simulink model "asbdhc2"  (Simulink 8.0)
settings: Solver=ode45  StartTime=0.0  StopTime=1000  MaxStep=1/30  RelTol=1e-2  AbsTol=1e-3
PreLoadFcn:
  | load asbdhc2_init;
values from neighbouring files (symbols this model uses):
  beaver_b = 14.63    [beaver_4_14_2013.mat]    (also in modelScript.m = 1.4224; monteCarloSim01.mat = 1.4224; simData_12_10_2013.mat = 1.4224; simData_12_9_2013.mat = 1.4224)
  beaver_c = 1.5875    [beaver_4_14_2013.mat]    (also in modelScript.m = 0.3302; monteCarloSim01.mat = 0.3302; simData_12_10_2013.mat = 0.3302; simData_12_9_2013.mat = 0.3302)
  beaver_init_p = 0    [beaver_4_14_2013.mat]    (also in monteCarloSim01.mat; simData_12_10_2013.mat; simData_12_9_2013.mat; simData_4_23_2013.mat)
  beaver_init_pitch = 0.13029612885    [beaver_4_14_2013.mat]    (also in monteCarloSim01.mat; simData_12_10_2013.mat; simData_12_9_2013.mat; simData_4_23_2013.mat)
  beaver_init_q = 0    [beaver_4_14_2013.mat]    (also in monteCarloSim01.mat; simData_12_10_2013.mat; simData_12_9_2013.mat; simData_4_23_2013.mat)
  beaver_init_r = 0    [beaver_4_14_2013.mat]    (also in monteCarloSim01.mat; simData_12_10_2013.mat; simData_12_9_2013.mat; simData_4_23_2013.mat)
  beaver_init_roll = 0    [beaver_4_14_2013.mat]    (also in monteCarloSim01.mat; simData_12_10_2013.mat; simData_12_9_2013.mat; simData_4_23_2013.mat)
  beaver_mass = 2288.231    [beaver_4_14_2013.mat]    (also in modelScript.m = 1.56; monteCarloSim01.mat = 1.56; simData_12_10_2013.mat = 1.56; simData_12_9_2013.mat = 1.56)
  beaver_S = 23.23    [beaver_4_14_2013.mat]    (also in modelScript.m = 0.2589; monteCarloSim01.mat = 0.2589; simData_12_10_2013.mat = 0.2589; simData_12_9_2013.mat = 0.2589)
  CD0 = 0.03    [modelScript.m]    (also in monteCarloSim01.mat; polarFun.m = x(1); simData_12_10_2013.mat; simData_12_9_2013.mat)
  Cl0 = 0.000591    [beaver_4_14_2013.mat]    (also in monteCarloSim01.mat; simData_12_10_2013.mat; simData_12_9_2013.mat; simData_4_23_2013.mat)
  Cl_alpha2_dpt = -0.01406    [beaver_4_14_2013.mat]    (also in monteCarloSim01.mat; simData_12_10_2013.mat; simData_12_9_2013.mat; simData_4_23_2013.mat)
  Cl_beta = -0.0618    [beaver_4_14_2013.mat]    (also in monteCarloSim01.mat; simData_12_10_2013.mat; simData_12_9_2013.mat; simData_4_23_2013.mat)
  Cl_da = -0.09917    [beaver_4_14_2013.mat]    (also in monteCarloSim01.mat; simData_12_10_2013.mat; simData_12_9_2013.mat; simData_4_23_2013.mat)
  Cl_da_alpha = -0.08269    [beaver_4_14_2013.mat]    (also in monteCarloSim01.mat; simData_12_10_2013.mat; simData_12_9_2013.mat; simData_4_23_2013.mat)
  Cl_dr = 0.006934    [beaver_4_14_2013.mat]    (also in monteCarloSim01.mat; simData_12_10_2013.mat; simData_12_9_2013.mat; simData_4_23_2013.mat)
  Cl_p = -0.5045    [beaver_4_14_2013.mat]    (also in monteCarloSim01.mat; simData_12_10_2013.mat; simData_12_9_2013.mat; simData_4_23_2013.mat)
  Cl_r = 0.1695    [beaver_4_14_2013.mat]    (also in monteCarloSim01.mat; simData_12_10_2013.mat; simData_12_9_2013.mat; simData_4_23_2013.mat)
  Cm0 = 0.09448    [beaver_4_14_2013.mat]    (also in monteCarloSim01.mat; simData_12_10_2013.mat; simData_12_9_2013.mat; simData_4_23_2013.mat)
  Cm_alpha = -0.6028    [beaver_4_14_2013.mat]    (also in monteCarloSim01.mat; simData_12_10_2013.mat; simData_12_9_2013.mat; simData_4_23_2013.mat)
  Cm_alpha2 = -2.14    [beaver_4_14_2013.mat]    (also in monteCarloSim01.mat; simData_12_10_2013.mat; simData_12_9_2013.mat; simData_4_23_2013.mat)
  Cm_beta2 = 0.6921    [beaver_4_14_2013.mat]    (also in monteCarloSim01.mat; simData_12_10_2013.mat; simData_12_9_2013.mat; simData_4_23_2013.mat)
  Cm_de = -1.921    [beaver_4_14_2013.mat]    (also in monteCarloSim01.mat; simData_12_10_2013.mat; simData_12_9_2013.mat; simData_4_23_2013.mat)
  Cm_df = 0.4072    [beaver_4_14_2013.mat]    (also in monteCarloSim01.mat; simData_12_10_2013.mat; simData_12_9_2013.mat; simData_4_23_2013.mat)
  Cm_dpt = -0.07895    [beaver_4_14_2013.mat]    (also in monteCarloSim01.mat; simData_12_10_2013.mat; simData_12_9_2013.mat; simData_4_23_2013.mat)
  Cm_q = -15.56    [beaver_4_14_2013.mat]    (also in monteCarloSim01.mat; simData_12_10_2013.mat; simData_12_9_2013.mat; simData_4_23_2013.mat)
  Cm_r = -0.3118    [beaver_4_14_2013.mat]    (also in monteCarloSim01.mat; simData_12_10_2013.mat; simData_12_9_2013.mat; simData_4_23_2013.mat)
  Cn0 = -0.003117    [beaver_4_14_2013.mat]    (also in monteCarloSim01.mat; simData_12_10_2013.mat; simData_12_9_2013.mat; simData_4_23_2013.mat)
  Cn_beta = 0.006719    [beaver_4_14_2013.mat]    (also in monteCarloSim01.mat; simData_12_10_2013.mat; simData_12_9_2013.mat; simData_4_23_2013.mat)
  Cn_beta3 = 0.1373    [beaver_4_14_2013.mat]    (also in monteCarloSim01.mat; simData_12_10_2013.mat; simData_12_9_2013.mat; simData_4_23_2013.mat)
  Cn_da = -0.003872    [beaver_4_14_2013.mat]    (also in monteCarloSim01.mat; simData_12_10_2013.mat; simData_12_9_2013.mat; simData_4_23_2013.mat)
  Cn_dpt3 = -0.003026    [beaver_4_14_2013.mat]    (also in monteCarloSim01.mat; simData_12_10_2013.mat; simData_12_9_2013.mat; simData_4_23_2013.mat)
  Cn_dr = -0.08265    [beaver_4_14_2013.mat]    (also in monteCarloSim01.mat; simData_12_10_2013.mat; simData_12_9_2013.mat; simData_4_23_2013.mat)
  Cn_p = -0.1585    [beaver_4_14_2013.mat]    (also in monteCarloSim01.mat; simData_12_10_2013.mat; simData_12_9_2013.mat; simData_4_23_2013.mat)
  Cn_q = 0.1595    [beaver_4_14_2013.mat]    (also in monteCarloSim01.mat; simData_12_10_2013.mat; simData_12_9_2013.mat; simData_4_23_2013.mat)
  Cn_r = -0.1112    [beaver_4_14_2013.mat]    (also in monteCarloSim01.mat; simData_12_10_2013.mat; simData_12_9_2013.mat; simData_4_23_2013.mat)
  Cx0 = -0.03554    [beaver_4_14_2013.mat]    (also in modelScript.m = 0; monteCarloSim01.mat = 0; simData_12_10_2013.mat = 0; simData_12_9_2013.mat = 0)
  Cx_alpha = 0.00292    [beaver_4_14_2013.mat]    (also in modelScript.m = 0; monteCarloSim01.mat = 0; simData_12_10_2013.mat = 0; simData_12_9_2013.mat = 0)
  Cx_alpha2 = 5.459    [beaver_4_14_2013.mat]    (also in modelScript.m = 0; monteCarloSim01.mat = 0; simData_12_10_2013.mat = 0; simData_12_9_2013.mat = 0)
  Cx_alpha3 = -5.162    [beaver_4_14_2013.mat]    (also in modelScript.m = 0; monteCarloSim01.mat = 0; simData_12_10_2013.mat = 0; simData_12_9_2013.mat = 0)
  Cx_df = -0.09447    [beaver_4_14_2013.mat]    (also in modelScript.m = 0; monteCarloSim01.mat = 0; simData_12_10_2013.mat = 0; simData_12_9_2013.mat = 0)
  Cx_df_alpha = 1.106    [beaver_4_14_2013.mat]    (also in modelScript.m = 0; monteCarloSim01.mat = 0; simData_12_10_2013.mat = 0; simData_12_9_2013.mat = 0)
  Cx_dpt = 0.1161    [beaver_4_14_2013.mat]    (also in modelScript.m = 0; monteCarloSim01.mat = 0; simData_12_10_2013.mat = 0; simData_12_9_2013.mat = 0)
  Cx_dpt2_alpha = 0.1453    [beaver_4_14_2013.mat]    (also in modelScript.m = 0; monteCarloSim01.mat = 0; simData_12_10_2013.mat = 0; simData_12_9_2013.mat = 0)
  Cx_dr = 0.03412    [beaver_4_14_2013.mat]    (also in modelScript.m = 0; monteCarloSim01.mat = 0; simData_12_10_2013.mat = 0; simData_12_9_2013.mat = 0)
  Cx_q = -0.6748    [beaver_4_14_2013.mat]    (also in modelScript.m = 0; monteCarloSim01.mat = 0; simData_12_10_2013.mat = 0; simData_12_9_2013.mat = 0)
  Cy0 = -0.002226    [beaver_4_14_2013.mat]    (also in modelScript.m = 0; monteCarloSim01.mat = 0; simData_12_10_2013.mat = 0; simData_12_9_2013.mat = 0)
  Cy_beta = -0.7678    [beaver_4_14_2013.mat]    (also in modelScript.m = 0; monteCarloSim01.mat = 0; simData_12_10_2013.mat = 0; simData_12_9_2013.mat = 0)
  Cy_da = -0.02956    [beaver_4_14_2013.mat]    (also in modelScript.m = 0; monteCarloSim01.mat = 0; simData_12_10_2013.mat = 0; simData_12_9_2013.mat = 0)
  Cy_dr = 0.1158    [beaver_4_14_2013.mat]    (also in modelScript.m = 0; monteCarloSim01.mat = 0; simData_12_10_2013.mat = 0; simData_12_9_2013.mat = 0)
  Cy_dr_alpha = 0.5238    [beaver_4_14_2013.mat]    (also in modelScript.m = 0; monteCarloSim01.mat = 0; simData_12_10_2013.mat = 0; simData_12_9_2013.mat = 0)
  Cy_p = -0.124    [beaver_4_14_2013.mat]    (also in modelScript.m = 0; monteCarloSim01.mat = 0; simData_12_10_2013.mat = 0; simData_12_9_2013.mat = 0)
  Cy_r = 0.3666    [beaver_4_14_2013.mat]    (also in modelScript.m = 0; monteCarloSim01.mat = 0; simData_12_10_2013.mat = 0; simData_12_9_2013.mat = 0)
  Cz0 = -0.05504    [beaver_4_14_2013.mat]    (also in modelScript.m = 0; monteCarloSim01.mat = 0; simData_12_10_2013.mat = 0; simData_12_9_2013.mat = 0)
  Cz_alpha = -5.578    [beaver_4_14_2013.mat]    (also in modelScript.m = 0; monteCarloSim01.mat = 0; simData_12_10_2013.mat = 0; simData_12_9_2013.mat = 0)
  Cz_alpha3 = 3.442    [beaver_4_14_2013.mat]    (also in modelScript.m = 0; monteCarloSim01.mat = 0; simData_12_10_2013.mat = 0; simData_12_9_2013.mat = 0)
  Cz_de = -0.398    [beaver_4_14_2013.mat]    (also in modelScript.m = 0; monteCarloSim01.mat = 0; simData_12_10_2013.mat = 0; simData_12_9_2013.mat = 0)
  Cz_de_beta = -15.93    [beaver_4_14_2013.mat]    (also in modelScript.m = 0; monteCarloSim01.mat = 0; simData_12_10_2013.mat = 0; simData_12_9_2013.mat = 0)
  Cz_df = -1.377    [beaver_4_14_2013.mat]    (also in modelScript.m = 0; monteCarloSim01.mat = 0; simData_12_10_2013.mat = 0; simData_12_9_2013.mat = 0)
  Cz_df_alpha = -1.261    [beaver_4_14_2013.mat]    (also in modelScript.m = 0; monteCarloSim01.mat = 0; simData_12_10_2013.mat = 0; simData_12_9_2013.mat = 0)
  Cz_dpt = -0.1563    [beaver_4_14_2013.mat]    (also in modelScript.m = 0; monteCarloSim01.mat = 0; simData_12_10_2013.mat = 0; simData_12_9_2013.mat = 0)
  Cz_q = -2.988    [beaver_4_14_2013.mat]    (also in modelScript.m = 0; monteCarloSim01.mat = 0; simData_12_10_2013.mat = 0; simData_12_9_2013.mat = 0)
  Ix = .1147    (= 0.1147)    [modelScript.m]    (also in monteCarloSim01.mat; simData_12_10_2013.mat; simData_12_9_2013.mat; simData_4_26_2013.mat)
  Ixz = .0015    (= 0.0015)    [modelScript.m]    (also in monteCarloSim01.mat; simData_12_10_2013.mat; simData_12_9_2013.mat; simData_4_26_2013.mat)
  Iy = .0576    (= 0.0576)    [modelScript.m]    (also in monteCarloSim01.mat; simData_12_10_2013.mat; simData_12_9_2013.mat; simData_4_26_2013.mat)
  Iz = .1712    (= 0.1712)    [modelScript.m]    (also in monteCarloSim01.mat; simData_12_10_2013.mat; simData_12_9_2013.mat; simData_4_26_2013.mat)
  KCL2 = 1/(pi*.7*beaver_b/beaver_c)    [modelScript.m]    (also in monteCarloSim01.mat = 0.0493425392361; polarFun.m = x(2); simData_12_10_2013.mat = 0.0493425392361; simData_12_9_2013.mat = 0.0493425392361)
  m = state.W/g(1)    [plant.m]
  nonLinearCd = [0.025 0.0283582705905 0.0317165411809 0.0350748117714 0.0384330823618 0.0417913529523 0.0451496235427 0.0485078941332 0.0518661647236 0.0552244353141 0.0585827059046 0.061940976495 ... (1000 elements, 1x1000)]    [NACA0012Adam.mat]    (also in monteCarloSim01.mat; simData_12_10_2013.mat; simData_12_9_2013.mat; simData_4_23_2013.mat)
  nonLinearCl = [0 0.0485067508622 0.0970135017244 0.145520252587 0.194027003449 0.240505289572 0.286480266666 0.332455243759 0.378430220853 0.421875006681 0.463843622747 0.505812238814 ... (1000 elements, 1x1000)]    [NACA0012Adam.mat]    (also in monteCarloSim01.mat; simData_12_10_2013.mat; simData_12_9_2013.mat; simData_4_23_2013.mat)
  nonLinearWindAeroAlpha = [-3.14159265359 -3.13530317881 -3.12901370403 -3.12272422924 -3.11643475446 -3.11014527968 -3.1038558049 -3.09756633012 -3.09127685533 -3.08498738055 -3.07869790577 -3.07240843099 ... (1000 elements, 1x1000)]    [NACA0012Adam.mat]    (also in monteCarloSim01.mat; simData_12_10_2013.mat; simData_12_9_2013.mat; simData_4_23_2013.mat)
  q = state.eulerRates(:,2)    [eulerKalman.m]
  r = state.eulerRates(:,3)    [eulerKalman.m]
  sampleVec = [1/1000 0]    [modelScript.m]    (also in monteCarloSim01.mat = [0.0909090909091 0]; simData_12_10_2013.mat = [0.0909090909091 0]; simData_12_9_2013.mat = [0.001 0]; simData_4_26_2013.mat = [0.02 0])
  u0 = 100/3.28    (= 30.487804878)    [modelScript.m]    (also in monteCarloSim01.mat; simData_12_10_2013.mat; simData_12_9_2013.mat; simData_4_26_2013.mat)
  uaero0 = [-0.0317656979071 -0.0320210159663 -0.0365180369264 0]    [beaver_4_14_2013.mat]    (also in monteCarloSim01.mat; simData_12_10_2013.mat; simData_12_9_2013.mat; simData_4_23_2013.mat)
  v0 = 0    [modelScript.m]    (also in monteCarloSim01.mat; simData_12_10_2013.mat; simData_12_9_2013.mat; simData_4_26_2013.mat)
  w0 = 0    [modelScript.m]    (also in monteCarloSim01.mat; simData_12_10_2013.mat; simData_12_9_2013.mat; simData_4_26_2013.mat)
undefined symbols (not defined in the file or in its folder): Earth, F, Light, MIL, s, sigbuilder_block, WGS84
libraries: aerolibconvert2 x5, aerolibtransform2 x4, aerolibadynsys x3, aerolibasang x3, aerolibwind2 x3, aerolibfltsims x3, aerolibanimutils x2, aerolib6dof2 x1, aerolibnav x1, aerolibutil x1, aerolibatmos2 x1, aerolibgravity2 x1
(part 1 of 2)
Description:
  | Fly the DeHavilland Beaver
  | 
  | This demonstration uses a pilot's joystick to allow you to fly the DeHavilland
  | Beaver modeled with Simulink(R), and Aerospace Blockset(TM) software.  This model has been
  | color coded to aid in locating Aerospace Blockset blocks. The red blocks are
  | Aerospace Blockset blocks, the orange blocks are subsystems containing
  | additional Aerospace Blockset blocks and the white blocks are Simulink blocks.
  | 
  | The DeHavilland Beaver model includes the airframe dynamics, including
  | aerodynamics. Effects of the environment are also modeled, such as wind profiles
  | for the landing phase. Visualization for this model is done via an interface to
  | FlightGear, a open source flight simulator package.
  | 
  | The DeHavilland Beaver was first flown in 1947. Today it is still prized by pilots
  | for its reliability and versatility. The DeHavilland Beaver can be operated on wheels,
  | skis or float landing gear.
  | 
  | Speed Max       110 kts
  | Altitude Max 10,000 ft
  | Range Max       400 nm
  | Load                     6 passengers
  | Crew                     1 member
  | 
  | For more information on the FlightGear interface, see the documentation.
settings Model: Creator=The MathWorks Inc.  LastModifiedBy=mufasa  ExtModeTrigMode=oneshot  ExtModeArmWhenConnect=off  ExtModeAutoUpdateStatusClock=off
settings DataIOCC: LimitDataPoints=off  SignalLoggingSaveFormat=ModelDataLogs  SignalLoggingName=sigsOut
settings OptimizationCC: InlineParams=on  InlineInvariantSignals=on  InitFltsAndDblsToZero=on  EfficientFloat2IntCast=on  EfficientMapNaN2IntZero=off
settings DebuggingCC: SolverPrmCheckMsg=none  MultiTaskDSMMsg=warning  MultiTaskCondExecSysMsg=none  SigSpecEnsureSampleTimeMsg=none  IntegerOverflowMsg=none  FcnCallInpInsideContextMsg=UseLocalSettings
settings HardwareCC: TargetEndianess=LittleEndian  TargetHWDeviceType=MATLAB Host  ProdEqTarget=off
settings RTWCC: IncludeERTFirstTime=on
settings GRTTargetCC: TargetFcnLib=ansi_tfl_tmw.mat  CombineOutputUpdateFcns=off  GRTInterface=on

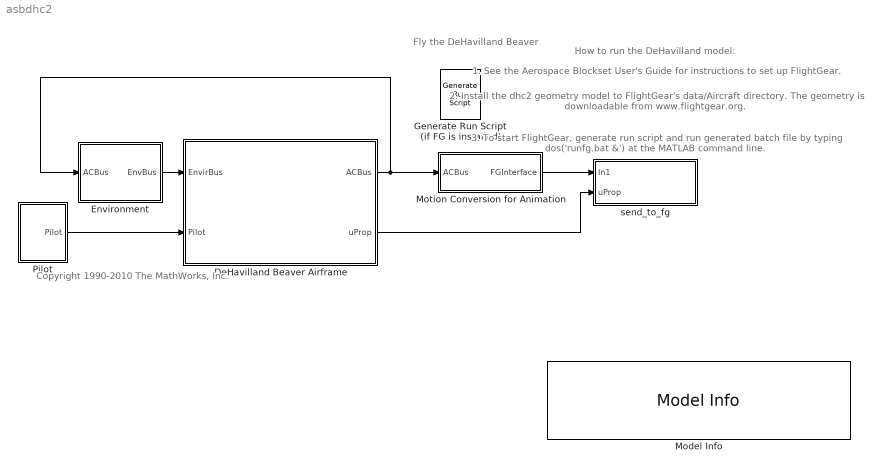
== system asbdhc2 ==
  note: 1. See the Aerospace Blockset User's Guide for instructions
      |     to set up FlightGear.
  note: Copyright 1990-2010 The MathWorks, Inc.
  note: Fly the DeHavilland Beaver
  note: 2. Install the dhc2 geometry model to FlightGear's data/Aircraft
      |     directory. The geometry is downloadable from www.flightgear.org.
  note: 3. To start FlightGear, generate run script and run generated batch
      |     file by typing dos('runfg.bat &') at the MATLAB command line.
  note: How to run the DeHavilland model:
  DeHavilland Beaver Airframe : Subsystem
      mask Display: image(imread('asbbeaver.jpg'))
  Environment : Subsystem
  Generate Run Script (if FG is installed) : aerolibfltsims/Generate Run Script  OutputFileName=runfg.bat  FlightGearBaseDirectory=C:\Program Files\FlightGear  GeometryModelName=dhc2F  DestinationPort=5502  OriginAddress=127.0.0.1  OriginPort=5505  LocalAddress=127.0.0.1  AirportId=KSFO  RunwayId=10L  InitialAltitude=7224  InitialHeading=113  OffsetDistance=4.72  OffsetAzimuth=0  GenerateFile=off  Architecture=Default  dataFlow=Send
  Model Info : simulink/Model-Wide Utilities/Model Info  InitialBlockCM=none  BlockCM=none  Frame=on  DisplayStringWithTags=|  HorizontalTextAlignment=Center  LeftAlignmentValue=0.5  SourceBlockDiagram=asbdhc2  TagMaxNumber=20
      | DeHavilland Beaver model 
      | %<ModelVersion>
      | Based on original work created by
      | Marc Rauw for Delft University of Technology 
      | http://www.dutchroll.com
  Motion Conversion for Animation : Subsystem
      mask Display:
      | port_label('input',1,'ACBus')
      | port_label('output',1,'\lambda,L,h,\phi,\theta,\psi','texmode','on')
  Pilot : Subsystem
  send_to_fg : Subsystem
  wires:
  DeHavilland Beaver Airframe/1(ACBus) -> Motion Conversion for Animation/1(ACBus), Environment/1(ACBus)
  Pilot/1(Pilot) -> DeHavilland Beaver Airframe/2(Pilot)
  Environment/1(EnvBus) -> DeHavilland Beaver Airframe/1(EnvirBus)
  Motion Conversion for Animation/1(FGInterface) -> send_to_fg/1(In1)
  DeHavilland Beaver Airframe/2(uProp) -> send_to_fg/2(uProp)

== system asbdhc2/DeHavilland Beaver Airframe ==
  EnvirBus : Inport
  Pilot : Inport  Port=2
  Aircraft Dynamics : Subsystem
  Calculate Parameters : Subsystem
  ACBus : Outport
  uProp : Outport  Port=2
  wires:
  Pilot/1 -> Aircraft Dynamics/1(Pilot)
  Aircraft Dynamics/1(AC Bus) -> Calculate Parameters/2(ACBus), ACBus/1
  EnvirBus/1 -> Aircraft Dynamics/2(EnvirBus), Calculate Parameters/1(EnvirBus)
  Calculate Parameters/1(FltParams) -> Aircraft Dynamics/3(FltParams)
  Aircraft Dynamics/2(uProp) -> uProp/1

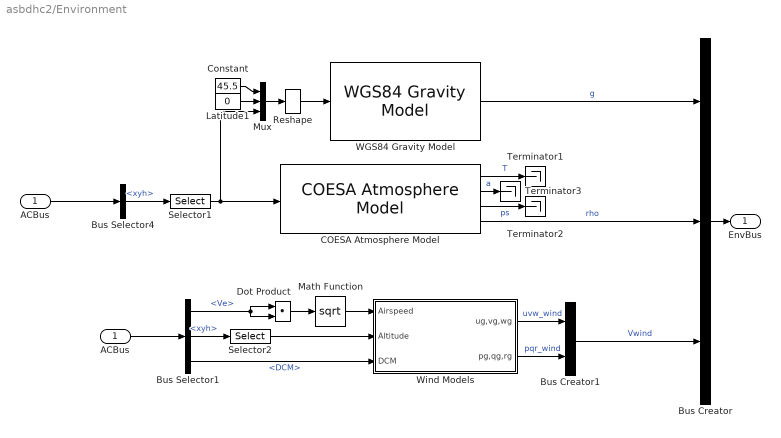
== system asbdhc2/Environment ==
  ACBus : Inport
  "ACBus " : InportShadow
  Bus Creator : BusCreator  Inputs=3
  Bus Creator1 : BusCreator  Inputs=2
  Bus Selector1 : BusSelector  OutputSignals=Ve,xyh,DCM
  Bus Selector4 : BusSelector  OutputSignals=xyh
  COESA Atmosphere Model : aerolibatmos2/COESA Atmosphere Model  units=Metric (MKS)  spec=1976 COESA-extended U.S. Standard Atmosphere  model=Profile  profile_var=High temperature  profile_percent=1%  profile_alt=5 km (16404 ft)  envelope_var=High temperature  envelope_percent=1%  action=Warning
  Constant : Constant  Value=45.5
  Dot Product : DotProduct  InputSameDT=on  OutDataTypeStr=Inherit: Inherit via internal rule
  Latitude1 : Constant  Value=0
  Math Function : Math  Operator=sqrt  SaturateOnIntegerOverflow=on
  Mux : Mux  Inputs=3
  Reshape : Reshape  OutputDimensionality=Row vector (2-D)
  Selector1 : Selector  InputPortWidth=3  IndexOptions=Index vector (dialog)  Indices=[3]  OutputSizes=1
  Selector2 : Selector  InputPortWidth=3  IndexOptions=Index vector (dialog)  Indices=[3]  OutputSizes=1
  Terminator1 : Terminator
  Terminator2 : Terminator
  Terminator3 : Terminator
  "WGS84 Gravity Model " : aerolibgravity2/WGS84 Gravity Model   model=WGS84 Taylor Series  units=Metric (MKS)  no_atmos=on  precessing=on  jd_loc=off  month=October  day=10  year=2004  no_centrifugal=on  action=None
  Wind Models : Subsystem
  EnvBus : Outport
  wires:
  COESA Atmosphere Model/4 -> Bus Creator/2  "rho"
  COESA Atmosphere Model/1 -> Terminator1/1  "T"
  COESA Atmosphere Model/3 -> Terminator2/1  "ps"
  COESA Atmosphere Model/2 -> Terminator3/1  "a"
  Selector1/1 -> COESA Atmosphere Model/1, Mux/3
  Bus Selector1/3 -> Wind Models/3(DCM)  "<DCM>"
  Wind Models/2(pg,qg,rg) -> Bus Creator1/2  "pqr_wind"
  Wind Models/1(ug,vg,wg) -> Bus Creator1/1  "uvw_wind"
  Bus Creator1/1 -> Bus Creator/3  "Vwind"
  Dot Product/1 -> Math Function/1
  Math Function/1 -> Wind Models/1(Airspeed)
  Bus Creator/1 -> EnvBus/1
  ACBus/1 -> Bus Selector4/1
  Bus Selector4/1 -> Selector1/1  "<xyh>"
  "ACBus "/1 -> Bus Selector1/1
  Bus Selector1/2 -> Selector2/1  "<xyh>"
  Selector2/1 -> Wind Models/2(Altitude)
  Bus Selector1/1 -> Dot Product/1, Dot Product/2  "<Ve>"
  Constant/1 -> Mux/1
  Latitude1/1 -> Mux/2
  Mux/1 -> Reshape/1
  "WGS84 Gravity Model "/1 -> Bus Creator/1  "g"
  Reshape/1 -> "WGS84 Gravity Model "/1

== system asbdhc2/Motion Conversion for Animation ==
  ACBus : Inport
  Angle Conversion : aerolibconvert2/Angle Conversion  IU=deg  OU=rad
  Bus Selector : BusSelector  OutputSignals=phi_theta_psi,Hdot,Ve,pqr,Vbody,bodyAccels
  Bus Selector1 : BusSelector  OutputSignals=Xe  OutputAsBus=on
  Constant : Constant  Value=0
  Flat Earth to LLA : aerolibtransform2/Flat Earth to LLA  units=Metric (MKS)  ptype=Earth (WGS84)  F=1/298.257223563  R=6378137  LL0=[37.6272 -122.3896]  psi=0
  Mux : Mux  Inputs=2
  Mux1 : Mux  Inputs=7
  Selector : Selector  InputPortWidth=2  IndexOptions=Index vector (dialog)  Indices=[2 1]  OutputSizes=1
  FGInterface : Outport
  wires:
  Mux1/1 -> FGInterface/1
  Constant/1 -> Flat Earth to LLA/2
  Bus Selector/1 -> Mux1/2  "<phi_theta_psi>"
  Mux/1 -> Mux1/1
  Flat Earth to LLA/2 -> Mux/2
  Flat Earth to LLA/1 -> Angle Conversion/1
  Bus Selector1/1 -> Flat Earth to LLA/1
  ACBus/1 -> Bus Selector/1, Bus Selector1/1
  Selector/1 -> Mux/1
  Bus Selector/2 -> Mux1/3  "<Hdot>"
  Bus Selector/3 -> Mux1/4  "<Ve>"
  Bus Selector/4 -> Mux1/5  "<pqr>"
  Bus Selector/5 -> Mux1/6  "<Vbody>"
  Bus Selector/6 -> Mux1/7  "<bodyAccels>"
  Angle Conversion/1 -> Selector/1

== system asbdhc2/Pilot ==
  Bus Creator : BusCreator  Inputs=2
  Flap : Subsystem  Tag=STV Subsys  LoadFcn=sigbuilder_block('load');  StartFcn=sigbuilder_block('start');  StopFcn=sigbuilder_block('stop');  ClipboardFcn=sigbuilder_block('clipboard');  mask(Sigbuilder block){}
      mask help: Sigbuilder GUI
      mask init:
      | if ~strcmp(get_param(bdroot(gcb),'SimulationStatus'),'stopped') tuvar = sigbuilder_block('maskInit'); end
      settings: CopyFcn=sigbuilder_block('copy');  DeleteFcn=sigbuilder_block('delete');  ModelCloseFcn=sigbuilder_block('modelClose');  PreSaveFcn=sigbuilder_block('preSave');  PauseFcn=sigbuilder_block('pause')  ContinueFcn=sigbuilder_block('continue')  NameChangeFcn=sigbuilder_block('namechange');  OpenFcn=sigbuilder_block('open',[127.5 251.25 511.5 271.5 ]);  CloseFcn=sigbuilder_block('close');
      mask Display: plot(0,0,100,100,[10,10,40,40,10],[80,20,20,80,80],[40,10],[50,50], [40,27,10],[65,72,56],[40,25,25,10],[28,28,43,43]);
  Input Signal  Conditioning : Subsystem
  Mux2 : Mux  Inputs=3
  Pilot Joystick : aerolibanimutils/Pilot Joystick  JoystickID=Joystick1  OutputConfiguration=FourAxis  SampleTime=1/30
  Rate Transition1 : RateTransition  OutPortSampleTime=0
  Rate Transition2 : RateTransition  OutPortSampleTime=0
  Pilot : Outport
  wires:
  Flap/1(Flap) -> Input Signal  Conditioning/3(Flap)
  Rate Transition1/1 -> Input Signal  Conditioning/1(Stick / Throt)
  Rate Transition2/1 -> Input Signal  Conditioning/2(Rudder)
  Input Signal  Conditioning/1(uaero) -> Bus Creator/1  "uaero"
  Input Signal  Conditioning/2(uprop) -> Bus Creator/2  "uprop"
  Bus Creator/1 -> Pilot/1
  Mux2/1 -> Rate Transition1/1
  Pilot Joystick/1 -> Mux2/1
  Pilot Joystick/3 -> Rate Transition2/1
  Pilot Joystick/4 -> Mux2/3
  Pilot Joystick/2 -> Mux2/2

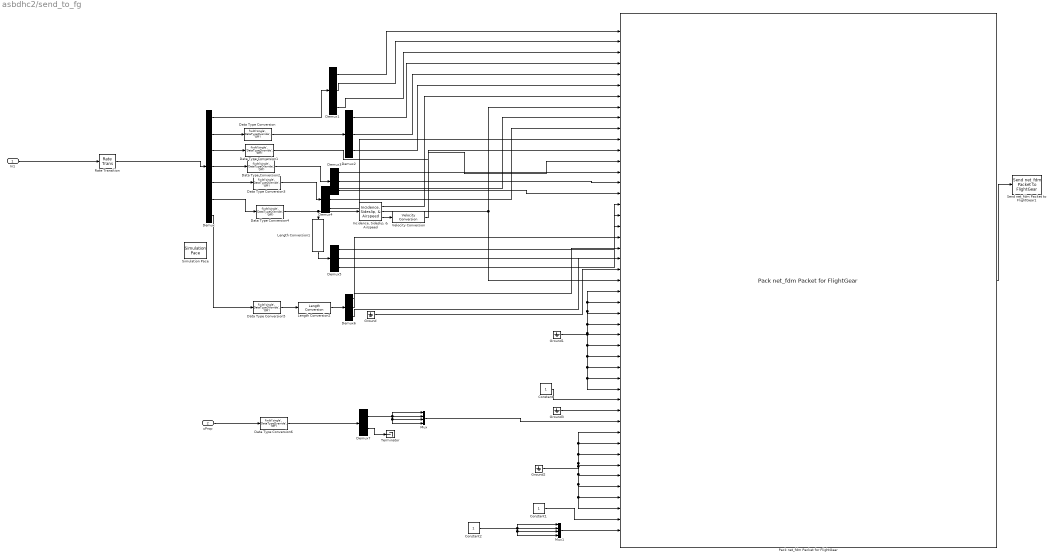
== system asbdhc2/send_to_fg ==
  In1 : Inport  OutDataTypeStr=double
  uProp : Inport  Port=2  OutDataTypeStr=double
  Constant : Constant  OutDataTypeStr=uint32
  Constant1 : Constant  OutDataTypeStr=fixdt('uint32', 'DataTypeOverride', 'Off')
  Constant2 : Constant  OutDataTypeStr=single
  Data Type Conversion{,1..6} (7 alike) : DataTypeConversion  OutDataTypeStr=fixdt('single', 'DataTypeOverride', 'Off')
  Demux : Demux  Outputs=7
  Demux{1..6} (6 alike) : Demux  Outputs=3
  Demux7 : Demux  Outputs=2
  Ground{,1..3} (4 alike) : Ground
  "Incidence, Sideslip, & Airspeed" : aerolibasang/Incidence, Sideslip, & Airspeed
  Length Conversion1 : aerolibconvert2/Length Conversion  IU=m  OU=ft
  Length Conversion2 : aerolibconvert2/Length Conversion  IU=m  OU=ft
  Mux : Mux
  Mux1 : Mux
  Pack net_fdm Packet for FlightGear : aerolibfltsims/Pack net_fdm Packet for FlightGear  FlightGearVersion=v2.0  ShowPositionAttitudeInputs=on  ShowVelocityAccelerationInputs=on  ShowControlSurfacePositionInputs=on  ShowEngineFuelInputs=on  ShowLandingGearInputs=off  ShowEnvironmentInputs=off  SampleTime=1/30
  Rate Transition : RateTransition  Integrity=off  Deterministic=off  OutPortSampleTime=1/30
  Send net_fdm Packet to FlightGear1 : aerolibfltsims/Send net_fdm Packet to FlightGear  DestinationIpAddress=127.0.0.1  DestinationPort=5502  LocalIpPort=-1  varLen=off  SampleTime=1/30
  Simulation Pace : aerolibanimutils/Simulation Pace  SimulationPace=1  SleepMode=MATLAB Thread  OutputPaceError=off  SampleTime=1/30
      settings: AttributesFormatString=%<SimulationPace> sec/sec
  Terminator : Terminator
  Velocity Conversion : aerolibconvert2/Velocity Conversion  IU=m/s  OU=kts
  wires:
  In1/1 -> Rate Transition/1
  Demux/1 -> Demux1/1
  Demux1/1 -> Pack net_fdm Packet for FlightGear/1
  Demux1/2 -> Pack net_fdm Packet for FlightGear/2
  Demux1/3 -> Pack net_fdm Packet for FlightGear/3
  Demux/2 -> Data Type Conversion/1
  Demux2/1 -> Pack net_fdm Packet for FlightGear/4
  Demux2/2 -> Pack net_fdm Packet for FlightGear/5
  Demux2/3 -> Pack net_fdm Packet for FlightGear/6
  Demux/6 -> Data Type Conversion4/1
  "Incidence, Sideslip, & Airspeed"/1 -> Pack net_fdm Packet for FlightGear/7
  "Incidence, Sideslip, & Airspeed"/2 -> Pack net_fdm Packet for FlightGear/8, Pack net_fdm Packet for FlightGear/24
  "Incidence, Sideslip, & Airspeed"/3 -> Velocity Conversion/1
  Demux/4 -> Data Type Conversion2/1
  Demux3/1 -> Pack net_fdm Packet for FlightGear/14
  Demux3/2 -> Pack net_fdm Packet for FlightGear/15
  Demux3/3 -> Pack net_fdm Packet for FlightGear/16
  Demux4/1 -> Pack net_fdm Packet for FlightGear/9
  Demux4/2 -> Pack net_fdm Packet for FlightGear/10
  Demux/5 -> Data Type Conversion3/1
  Ground/1 -> Pack net_fdm Packet for FlightGear/23
  Demux5/1 -> Pack net_fdm Packet for FlightGear/17
  Demux5/2 -> Pack net_fdm Packet for FlightGear/18
  Demux5/3 -> Pack net_fdm Packet for FlightGear/19
  Demux/7 -> Data Type Conversion5/1
  Demux6/1 -> Pack net_fdm Packet for FlightGear/20
  Demux6/2 -> Pack net_fdm Packet for FlightGear/21
  Demux6/3 -> Pack net_fdm Packet for FlightGear/22
  Rate Transition/1 -> Demux/1
  Pack net_fdm Packet for FlightGear/1 -> Send net_fdm Packet to FlightGear1/1
  Demux4/3 -> Pack net_fdm Packet for FlightGear/11
  Demux/3 -> Data Type Conversion1/1
  Data Type Conversion/1 -> Demux2/1
  Data Type Conversion1/1 -> Pack net_fdm Packet for FlightGear/13
  Data Type Conversion2/1 -> Demux3/1
  Data Type Conversion3/1 -> Demux4/1
  Data Type Conversion4/1 -> "Incidence, Sideslip, & Airspeed"/1, Length Conversion1/1
  Data Type Conversion5/1 -> Length Conversion2/1
  Velocity Conversion/1 -> Pack net_fdm Packet for FlightGear/12
  Length Conversion1/1 -> Demux5/1
  Length Conversion2/1 -> Demux6/1
  Ground1/1 -> Pack net_fdm Packet for FlightGear/25, Pack net_fdm Packet for FlightGear/26, Pack net_fdm Packet for FlightGear/27, Pack net_fdm Packet for FlightGear/28, Pack net_fdm Packet for FlightGear/29, Pack net_fdm Packet for FlightGear/30, Pack net_fdm Packet for FlightGear/31, Pack net_fdm Packet for FlightGear/32, Pack net_fdm Packet for FlightGear/33, Pack net_fdm Packet for FlightGear/34
  Constant/1 -> Pack net_fdm Packet for FlightGear/35
  Ground2/1 -> Pack net_fdm Packet for FlightGear/38, Pack net_fdm Packet for FlightGear/39, Pack net_fdm Packet for FlightGear/40, Pack net_fdm Packet for FlightGear/41, Pack net_fdm Packet for FlightGear/42, Pack net_fdm Packet for FlightGear/43, Pack net_fdm Packet for FlightGear/44, Pack net_fdm Packet for FlightGear/45
  Ground3/1 -> Pack net_fdm Packet for FlightGear/36
  uProp/1 -> Data Type Conversion6/1
  Demux7/2 -> Terminator/1
  Demux7/1 -> Mux/1, Mux/2, Mux/3, Mux/4
  Mux/1 -> Pack net_fdm Packet for FlightGear/37
  Constant2/1 -> Mux1/1, Mux1/2, Mux1/3, Mux1/4
  Mux1/1 -> Pack net_fdm Packet for FlightGear/47
  Data Type Conversion6/1 -> Demux7/1
  Constant1/1 -> Pack net_fdm Packet for FlightGear/46

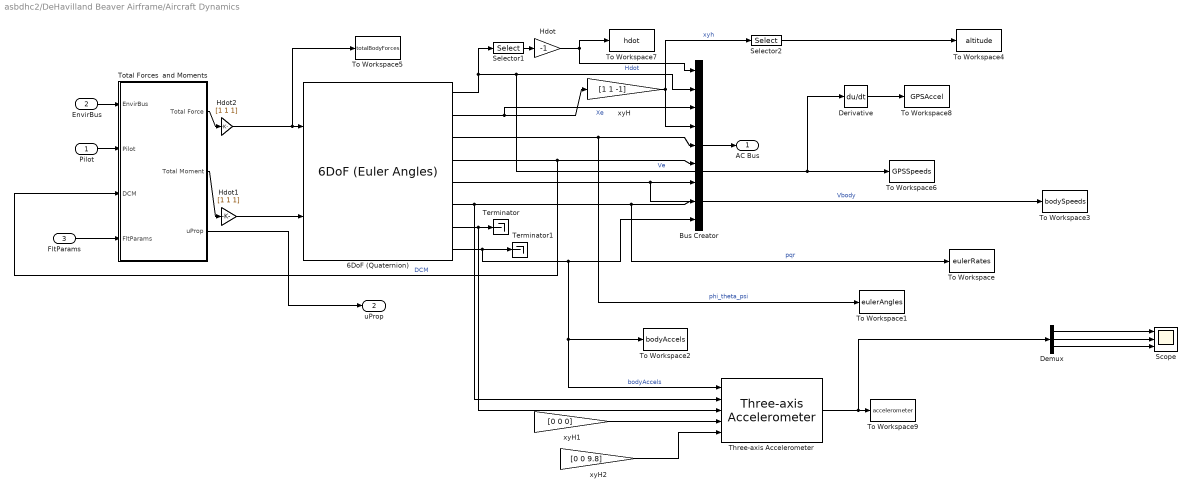
== system asbdhc2/DeHavilland Beaver Airframe/Aircraft Dynamics ==
  Pilot : Inport
  EnvirBus : Inport  Port=2
  FltParams : Inport  Port=3
  6DoF (Quaternion) : aerolib6dof2/6DoF (Euler Angles)  units=Metric (MKS)  mtype=Fixed  rep=Quaternion  xme_0=xme_0  Vm_0=[u0 v0 w0]  eul_0=[beaver_init_roll, beaver_init_pitch, 113/180*pi]  pm_0=[beaver_init_p, beaver_init_q, beaver_init_r]  mass_0=beaver_mass  mass_e=0  mass_f=0  inertia=[Ix 0 Ixz; 0 Iy 0; Ixz 0 Iz]  inertia_e=eye(3)  inertia_f=eye(3)  k_quat=1.0
  Bus Creator : BusCreator  Inputs=9
  Demux : Demux  Outputs=3
  Derivative : Derivative
  Hdot : Gain  Gain=-1  SaturateOnIntegerOverflow=on  OutDataTypeStr=Inherit: Same as input  ParamDataTypeStr=Inherit: Same as input
  Hdot1 : Gain  Gain=[1 1 1]  SaturateOnIntegerOverflow=on  OutDataTypeStr=Inherit: Same as input  ParamDataTypeStr=Inherit: Same as input
  Hdot2 : Gain  Gain=[1 1 1]  SaturateOnIntegerOverflow=on  OutDataTypeStr=Inherit: Same as input  ParamDataTypeStr=Inherit: Same as input
  Scope : Scope  NumInputPorts=3
      settings: TimeRange=10  YMin=-1~-1~-35  YMax=1~1~35
  Selector1 : Selector  InputPortWidth=3  IndexOptions=Index vector (dialog)  Indices=[3]  OutputSizes=1
  Selector2 : Selector  InputPortWidth=3  IndexOptions=Index vector (dialog)  Indices=[3]  OutputSizes=1
  Terminator : Terminator
  Terminator1 : Terminator
  Three-axis Accelerometer : aerolibnav/Three-axis Accelerometer  units=Metric (MKS)  acc=[0 0 0]  gtype=on  dtype_a=on  w_a=190  z_a=0.707  a_sf_cc=[1 0 0; 0 1 0; 0 0 1]  a_bias=[0 0 0]  a_rand=off  a_seeds=[23093 23094 23095]  a_pow=[0.001 0.001 0.001]  a_sat="[-inf  -inf  -inf  inf inf inf]"  a_Ts=0
  To Workspace : ToWorkspace  VariableName=eulerRates  SampleTime=sampleVec  SaveFormat=Structure With Time
  To Workspace1 : ToWorkspace  VariableName=eulerAngles  SampleTime=sampleVec  SaveFormat=Structure With Time
  To Workspace2 : ToWorkspace  VariableName=bodyAccels  SampleTime=sampleVec  SaveFormat=Structure With Time
  To Workspace3 : ToWorkspace  VariableName=bodySpeeds  SampleTime=sampleVec  SaveFormat=Structure With Time
  To Workspace4 : ToWorkspace  VariableName=altitude  SampleTime=-1  SaveFormat=Structure With Time
  To Workspace5 : ToWorkspace  VariableName=totalBodyForces  SampleTime=-1  SaveFormat=Structure With Time
  To Workspace6 : ToWorkspace  VariableName=GPSSpeeds  SampleTime=[1/5 0]  SaveFormat=Structure With Time
  To Workspace7 : ToWorkspace  VariableName=hdot  SampleTime=-1  SaveFormat=Structure With Time
  To Workspace8 : ToWorkspace  VariableName=GPSAccel  SampleTime=[1/50 0]  SaveFormat=Structure With Time
  To Workspace9 : ToWorkspace  VariableName=accelerometer  SampleTime=sampleVec  SaveFormat=Structure With Time
  Total Forces  and Moments : Subsystem
  xyH : Gain  Gain=[1 1 -1]  SaturateOnIntegerOverflow=on  OutDataTypeStr=Inherit: Same as input  ParamDataTypeStr=Inherit: Same as input
  xyH1 : Gain  Gain=[0 0 0]  SaturateOnIntegerOverflow=on  OutDataTypeStr=Inherit: Same as input  ParamDataTypeStr=Inherit: Same as input
  xyH2 : Gain  Gain=[0 0 9.8]  SaturateOnIntegerOverflow=on  OutDataTypeStr=Inherit: Same as input  ParamDataTypeStr=Inherit: Same as input
  AC Bus : Outport
  uProp : Outport  Port=2
  wires:
  6DoF (Quaternion)/4 -> Bus Creator/6, Total Forces  and Moments/3(DCM)  "DCM"
  6DoF (Quaternion)/3 -> Bus Creator/5, To Workspace1/1  "phi_theta_psi"
  6DoF (Quaternion)/2 -> xyH/1, Bus Creator/3  "Xe"
  6DoF (Quaternion)/5 -> Bus Creator/7, To Workspace3/1  "Vbody"
  6DoF (Quaternion)/7 -> Terminator/1, Three-axis Accelerometer/3
  6DoF (Quaternion)/1 -> Selector1/1, Bus Creator/2, To Workspace6/1, Derivative/1  "Ve"
  Pilot/1 -> Total Forces  and Moments/2(Pilot)
  Selector1/1 -> Hdot/1
  Total Forces  and Moments/1(Total Force) -> Hdot2/1
  Total Forces  and Moments/2(Total Moment) -> Hdot1/1
  xyH/1 -> Bus Creator/4, Selector2/1  "xyh"
  Hdot/1 -> Bus Creator/1, To Workspace7/1  "Hdot"
  6DoF (Quaternion)/8 -> Terminator1/1, Bus Creator/9, Three-axis Accelerometer/1, To Workspace2/1  "bodyAccels"
  Bus Creator/1 -> AC Bus/1
  EnvirBus/1 -> Total Forces  and Moments/1(EnvirBus)
  6DoF (Quaternion)/6 -> Three-axis Accelerometer/2, Bus Creator/8, To Workspace/1  "pqr"
  FltParams/1 -> Total Forces  and Moments/4(FltParams)
  Total Forces  and Moments/3(uProp) -> uProp/1
  Selector2/1 -> To Workspace4/1
  Derivative/1 -> To Workspace8/1
  Hdot1/1 -> 6DoF (Quaternion)/2
  Hdot2/1 -> 6DoF (Quaternion)/1, To Workspace5/1
  xyH1/1 -> Three-axis Accelerometer/4
  Demux/1 -> Scope/1
  Demux/2 -> Scope/2
  Demux/3 -> Scope/3
  Three-axis Accelerometer/1 -> Demux/1, To Workspace9/1
  xyH2/1 -> Three-axis Accelerometer/5

== system asbdhc2/DeHavilland Beaver Airframe/Calculate Parameters ==
  EnvirBus : Inport
  ACBus : Inport  Port=2
  "ACBus " : InportShadow  Port=2
  Bus Creator : BusCreator  Inputs=5
  Bus Selector1 : BusSelector  OutputSignals=rho
  Bus Selector2 : BusSelector  OutputSignals=Vbody
  Bus Selector3 : BusSelector  OutputSignals=pqr,Ve
  Bus Selector4 : BusSelector  OutputSignals=Vwind.uvw_wind,Vwind.pqr_wind
  Dynamic Pressure : aerolibasang/Dynamic Pressure
  "Incidence, Sideslip, & Airspeed" : aerolibasang/Incidence, Sideslip, & Airspeed
  Sum2 : Sum  Inputs=|++  SaturateOnIntegerOverflow=on  InputSameDT=on  OutDataTypeStr=Inherit: Same as first input
  Sum4 : Sum  Inputs=+-|  SaturateOnIntegerOverflow=on  InputSameDT=on  OutDataTypeStr=Inherit: Same as first input
  To Workspace : ToWorkspace  VariableName=rho  SampleTime=sampleVec  SaveFormat=Structure With Time
  FltParams : Outport
  wires:
  "ACBus "/1 -> Bus Selector2/1
  Bus Creator/1 -> FltParams/1
  Bus Selector3/1 -> Sum2/2  "<pqr>"
  ACBus/1 -> Bus Selector3/1
  Bus Selector1/1 -> Dynamic Pressure/2, To Workspace/1  "<rho>"
  EnvirBus/1 -> Bus Selector1/1, Bus Selector4/1
  Dynamic Pressure/1 -> Bus Creator/5  "Qdyn"
  Bus Selector3/2 -> Dynamic Pressure/1  "<Ve>"
  Bus Selector4/2 -> Sum2/1  "<pqr_wind>"
  Sum4/1 -> "Incidence, Sideslip, & Airspeed"/1
  "Incidence, Sideslip, & Airspeed"/1 -> Bus Creator/1  "alpha"
  "Incidence, Sideslip, & Airspeed"/2 -> Bus Creator/2  "beta"
  "Incidence, Sideslip, & Airspeed"/3 -> Bus Creator/3  "V"
  Bus Selector2/1 -> Sum4/1  "<Vbody>"
  Bus Selector4/1 -> Sum4/2  "<uvw_wind>"
  Sum2/1 -> Bus Creator/4  "pqr_tot"

== system asbdhc2/Environment/Wind Models ==
  Airspeed : Inport
  Altitude : Inport  Port=2
  DCM : Inport  Port=3
  "DCM " : InportShadow  Port=3
  Discrete Wind Gust Model : aerolibwind2/Discrete Wind Gust Model  units=Metric (MKS)  Gx=off  Gy=off  Gz=off  t_0=20  d_m=[120 120 80]  v_m=[3.5 3.5 3.0]
  Dryden Wind Turbulence Model  (Continuous (+q -r)) : aerolibwind2/Dryden Wind Turbulence Model  (Continuous (+q -r))  units=Metric (MKS)  spec=MIL-F-8785C  model=Continuous Dryden (+q -r)  W20=windSpeed  Wdeg=0  TurbProb=10^-2 - Light  L_high=533.4  Wingspan=beaver_b  ts=0.1  Seed=[23341 23342 23343 23344]  T_on=on
  Sum : Sum  Inputs=+++  SaturateOnIntegerOverflow=on  InputSameDT=on  OutDataTypeStr=Inherit: Same as first input
  Wind Shear Model : aerolibwind2/Wind Shear Model  units=Metric (MKS)  phase=Category C - Terminal Flight Phase  W_20=windSpeed  Wdeg=0
  ug,vg,wg : Outport
  pg,qg,rg : Outport  Port=2
  wires:
  "DCM "/1 -> Dryden Wind Turbulence Model  (Continuous (+q -r))/3
  Wind Shear Model/1 -> Sum/1
  Dryden Wind Turbulence Model  (Continuous (+q -r))/1 -> Sum/2
  Discrete Wind Gust Model/1 -> Sum/3
  Sum/1 -> ug,vg,wg/1
  DCM/1 -> Wind Shear Model/2
  Airspeed/1 -> Dryden Wind Turbulence Model  (Continuous (+q -r))/2, Discrete Wind Gust Model/1
  Dryden Wind Turbulence Model  (Continuous (+q -r))/2 -> pg,qg,rg/1
  Altitude/1 -> Dryden Wind Turbulence Model  (Continuous (+q -r))/1, Wind Shear Model/1

== system asbdhc2/Pilot/Flap ==
  Demux : Demux  Tag=STV Demux  Outputs=1
  FromWs : FromWorkspace  Tag=STV FromWs  VariableName=tuvar  SampleTime=0  OutputAfterFinalValue=Holding final value  SigBuilderData=DataTag0  VnvData=DataTag1
      SigBuilderData=|
      | dataSet.timeRange = [0 300]
      | dataSet.name = 'Group 1'
      | sbobj.Groups.Name = 'Group 1'
      | sbobj.Groups.Signals.Name = 'Flap'
      | sbobj.Groups.Signals.XData = [0 4 4 6 6 300]
      | sbobj.Groups.Signals.YData = [0 0 0 0 0 0]
      | sbobj.Groups.TimeRange = [0 300]
  Flap : Outport  Tag=STV Outport
  wires:
  Demux/1 -> Flap/1
  FromWs/1 -> Demux/1

== system asbdhc2/Pilot/Input Signal  Conditioning ==
  Stick / Throt : Inport
  Rudder : Inport  Port=2
  Flap : Inport  Port=3
  Angle Conversion5 : aerolibconvert2/Angle Conversion  IU=deg  OU=rad
  Look-Up Table : Lookup  InputValues=[0:3]  Table=[0 4 10 20]  SaturateOnIntegerOverflow=on
  Mux1 : Mux
  Mux2 : Mux  Inputs=2
  RPM2ManifoldPressure : Lookup_n-D  NumberOfTableDimensions=1  BreakpointsForDimension1=[0 1800 2300]  IndexSearchMethod=Linear search  BeginIndexSearchUsingPreviousIndexResult=on  Table=[0 22.5735 26]  ExtrapMethod=Clip  InputSameDT=on
  Rate Limiter : RateLimiter  RisingSlewLimit=0.5  FallingSlewLimit=-0.5
  Throttle2RPM : Lookup_n-D  NumberOfTableDimensions=1  BreakpointsForDimension1=(1/6)*(3+([-3:3]))  IndexSearchMethod=Linear search  BeginIndexSearchUsingPreviousIndexResult=on  Table=((1+tanh([-3:3]))/(1+tanh(2.65))-0.0025)*2300  ExtrapMethod=Clip  InputSameDT=on
  demux : Demux  Outputs=3
  flip sign : Gain  Gain=-25  SaturateOnIntegerOverflow=on  OutDataTypeStr=Inherit: Same as input  ParamDataTypeStr=Inherit: Same as input
  flip sign1 : Gain  Gain=-15  SaturateOnIntegerOverflow=on  OutDataTypeStr=Inherit: Same as input  ParamDataTypeStr=Inherit: Same as input
  flip sign2 : Gain  Gain=-20  SaturateOnIntegerOverflow=on  OutDataTypeStr=Inherit: Same as input  ParamDataTypeStr=Inherit: Same as input
  uaero : Outport
  uprop : Outport  Port=2
  wires:
  demux/3 -> Throttle2RPM/1
  Flap/1 -> Rate Limiter/1
  Rate Limiter/1 -> Look-Up Table/1
  Stick / Throt/1 -> demux/1
  Rudder/1 -> flip sign/1
  Look-Up Table/1 -> Mux1/4
  demux/1 -> flip sign1/1
  demux/2 -> flip sign2/1
  Mux1/1 -> Angle Conversion5/1
  Angle Conversion5/1 -> uaero/1
  RPM2ManifoldPressure/1 -> Mux2/2
  Mux2/1 -> uprop/1
  flip sign/1 -> Mux1/3
  Throttle2RPM/1 -> Mux2/1, RPM2ManifoldPressure/1
  flip sign1/1 -> Mux1/2
  flip sign2/1 -> Mux1/1

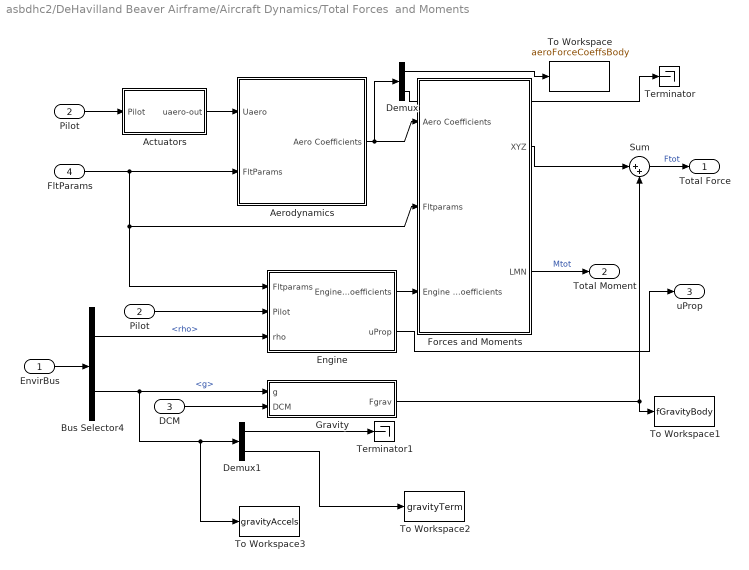
== system asbdhc2/DeHavilland Beaver Airframe/Aircraft Dynamics/Total Forces  and Moments ==
  EnvirBus : Inport
  Pilot : Inport  Port=2
  DCM : Inport  Port=3
  FltParams : Inport  Port=4
  Actuators : Subsystem
  Aerodynamics : Subsystem
  Bus Selector4 : BusSelector  OutputSignals=rho,g
  Demux : Demux  Outputs=[3 3]
  Demux1 : Demux  Outputs=[2 1]
  "Engine " : Subsystem
  Forces and Moments : Subsystem
  "Gravity " : Subsystem
  "Pilot " : InportShadow  Port=2
  Sum : Sum  Inputs=|++  SaturateOnIntegerOverflow=on  InputSameDT=on  OutDataTypeStr=Inherit: Same as first input
  Terminator : Terminator
  Terminator1 : Terminator
  To Workspace : ToWorkspace  VariableName=aeroForceCoeffsBody  SampleTime=-1  SaveFormat=Structure With Time
  To Workspace1 : ToWorkspace  VariableName=fGravityBody  SampleTime=sampleVec  SaveFormat=Structure With Time
  To Workspace2 : ToWorkspace  VariableName=gravityTerm  SampleTime=-1  SaveFormat=Structure With Time
  To Workspace3 : ToWorkspace  VariableName=gravityAccels  SampleTime=sampleVec  SaveFormat=Structure With Time
  Total Force : Outport
  Total Moment : Outport  Port=2
  uProp : Outport  Port=3
  wires:
  Forces and Moments/1(XYZ) -> Sum/1
  "Engine "/1(Engine Coefficients) -> Forces and Moments/3(Engine Coefficients)
  "Gravity "/1(Fgrav) -> Sum/2, To Workspace1/1
  Aerodynamics/1(Aero Coefficients) -> Forces and Moments/1(Aero Coefficients), Demux/1
  Pilot/1 -> Actuators/1(Pilot)
  Bus Selector4/1 -> "Engine "/3(rho)  "<rho>"
  DCM/1 -> "Gravity "/2(DCM)
  Bus Selector4/2 -> "Gravity "/1(g), To Workspace3/1, Demux1/1  "<g>"
  Sum/1 -> Total Force/1  "Ftot"
  Forces and Moments/2(LMN) -> Total Moment/1  "Mtot"
  "Pilot "/1 -> "Engine "/2(Pilot)
  FltParams/1 -> Forces and Moments/2(Fltparams), "Engine "/1(Fltparams), Aerodynamics/2(FltParams)
  Actuators/1(uaero-out) -> Aerodynamics/1(Uaero)
  EnvirBus/1 -> Bus Selector4/1
  "Engine "/2(uProp) -> uProp/1
  Demux/1 -> To Workspace/1
  Demux/2 -> Terminator/1
  Demux1/2 -> To Workspace2/1
  Demux1/1 -> Terminator1/1

== system asbdhc2/DeHavilland Beaver Airframe/Aircraft Dynamics/Total Forces  and Moments/Actuators ==
  Pilot : Inport
  Bus Selector2 : BusSelector  OutputSignals=uaero
  Demux : Demux
  Initial inputs for aero : Constant  Value=uaero0
  Mux : Mux
  Sum1 : Sum  Inputs=++|  SaturateOnIntegerOverflow=on  InputSameDT=on  OutDataTypeStr=Inherit: Same as first input
  uaero-out : Outport
  wires:
  Pilot/1 -> Bus Selector2/1
  Initial inputs for aero/1 -> Sum1/1
  Sum1/1 -> uaero-out/1
  Bus Selector2/1 -> Demux/1  "<uaero>"
  Demux/4 -> Mux/4
  Demux/1 -> Mux/1
  Demux/2 -> Mux/2
  Demux/3 -> Mux/3
  Mux/1 -> Sum1/2

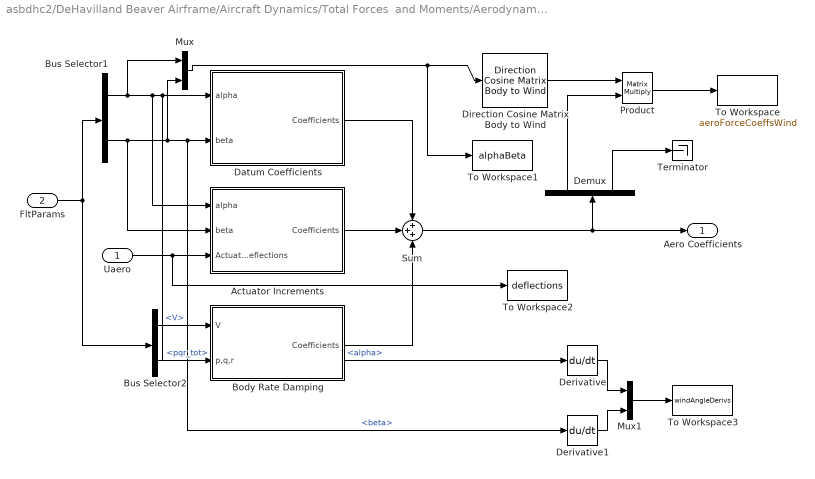
== system asbdhc2/DeHavilland Beaver Airframe/Aircraft Dynamics/Total Forces  and Moments/Aerodynamics ==
  Uaero : Inport
  FltParams : Inport  Port=2
  Actuator Increments : Subsystem
  Body Rate Damping : Subsystem
  Bus Selector1 : BusSelector  OutputSignals=alpha,beta
  Bus Selector2 : BusSelector  OutputSignals=V,pqr_tot
  Datum Coefficients : Subsystem
  Demux : Demux  Outputs=[3 3]
  Derivative : Derivative
  Derivative1 : Derivative
  Direction Cosine Matrix Body to Wind : aerolibtransform2/Direction Cosine Matrix Body to Wind
  Mux : Mux  Inputs=2
  Mux1 : Mux  Inputs=2
  Product : Product  Multiplication=Matrix(*)  RndMeth=Zero
  Sum : Sum  Inputs=+++  SaturateOnIntegerOverflow=on
  Terminator : Terminator
  To Workspace : ToWorkspace  VariableName=aeroForceCoeffsWind  SampleTime=-1  SaveFormat=Structure With Time
  To Workspace1 : ToWorkspace  VariableName=alphaBeta  SampleTime=sampleVec  SaveFormat=Structure
  To Workspace2 : ToWorkspace  VariableName=deflections  SampleTime=-1  SaveFormat=Structure With Time
  To Workspace3 : ToWorkspace  VariableName=windAngleDerivs  SampleTime=sampleVec  SaveFormat=Structure With Time
  Aero Coefficients : Outport
  wires:
  Bus Selector1/2 -> Actuator Increments/2(beta), Datum Coefficients/2(beta), Derivative1/1, Mux/2  "<beta>"
  Sum/1 -> Aero Coefficients/1, Demux/1
  Body Rate Damping/1(Coefficients) -> Sum/3
  Datum Coefficients/1(Coefficients) -> Sum/1
  Actuator Increments/1(Coefficients) -> Sum/2
  Bus Selector2/1 -> Body Rate Damping/1(V)  "<V>"
  Bus Selector2/2 -> Body Rate Damping/2(p,q,r)  "<pqr_tot>"
  Uaero/1 -> Actuator Increments/3(Actuator Deflections), To Workspace2/1
  Bus Selector1/1 -> Actuator Increments/1(alpha), Datum Coefficients/1(alpha), Derivative/1, Mux/1  "<alpha>"
  FltParams/1 -> Bus Selector1/1, Bus Selector2/1
  Mux/1 -> Direction Cosine Matrix Body to Wind/1, To Workspace1/1
  Direction Cosine Matrix Body to Wind/1 -> Product/1
  Product/1 -> To Workspace/1
  Demux/1 -> Product/2
  Demux/2 -> Terminator/1
  Derivative/1 -> Mux1/1
  Derivative1/1 -> Mux1/2
  Mux1/1 -> To Workspace3/1

== system asbdhc2/DeHavilland Beaver Airframe/Aircraft Dynamics/Total Forces  and Moments/Engine  ==
  Fltparams : Inport
  Pilot : Inport  Port=2
  rho : Inport  Port=3
  Bus Selector1 : BusSelector  OutputSignals=uprop
  Bus Selector4 : BusSelector  OutputSignals=V,alpha
  eng : Subsystem
  pow : Subsystem
  Engine Coefficients : Outport
  uProp : Outport  Port=2
  wires:
  Bus Selector4/1 -> pow/3(V)  "<V>"
  rho/1 -> pow/1(rho)
  Bus Selector4/2 -> eng/2(alpha)  "<alpha>"
  eng/1(Cprop) -> Engine Coefficients/1
  Pilot/1 -> pow/2(Pilot), Bus Selector1/1
  pow/1(dpt) -> eng/1(dpt)
  Fltparams/1 -> Bus Selector4/1
  Bus Selector1/1 -> uProp/1  "<uprop>"

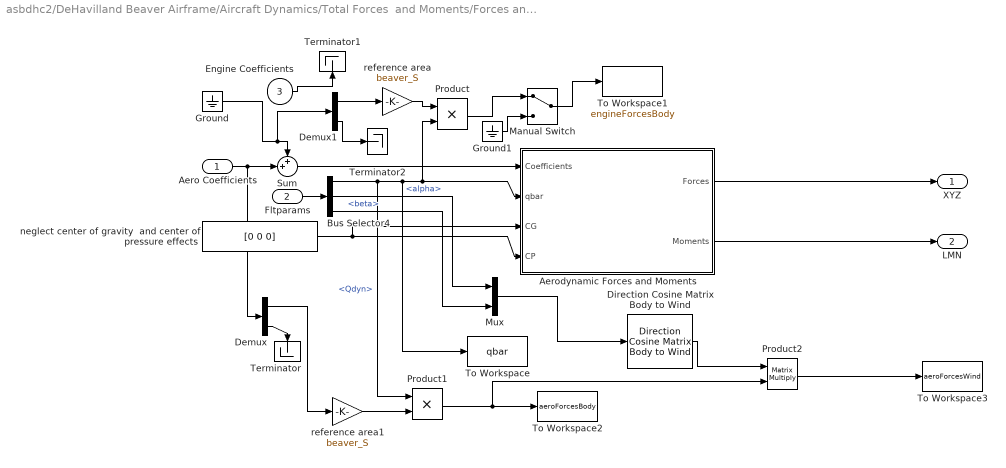
== system asbdhc2/DeHavilland Beaver Airframe/Aircraft Dynamics/Total Forces  and Moments/Forces and Moments ==
  Aero Coefficients : Inport
  Fltparams : Inport  Port=2
  Engine Coefficients : Inport  Port=3
  Aerodynamic Forces and Moments : Subsystem  AncestorBlock=aerolibadyn/Aerodynamic Forces and Moments  mask(Aerodynamic Forces and Moments){inputAxes=Body, outputForceAxes=Body, outputMomentAxes=Body, S=beaver_S, b=beaver_b, cbar=beaver_c}
      mask prompts: inputAxes "Input axes:"; outputForceAxes "Force axes:"; outputMomentAxes "Moment axes:"; S "Reference area:"; b "Reference span:"; cbar "Reference length:"
      mask help: Compute the aerodynamic forces and moments applied at the center of gravity using the aerodynamic coefficients, dynamic pressure, center of gravity and center of pressure.
      mask init:
      | ports=aeroicon('aeroblkadyn','icon');
      mask Help: eval('asbhelp');
      mask TypeOptions inputAxes: Body | Stability | Wind
      mask TypeOptions outputForceAxes: Body | Stability | Wind
      mask TypeOptions outputMomentAxes: Body | Stability | Wind
      mask Display:
      | port_label(ports(1).type,ports(1).port,ports(1).txt,'texmode','on');
      | port_label(ports(2).type,ports(2).port,ports(2).txt,'texmode','on');
      | port_label(ports(3).type,ports(3).port,ports(3).txt,'texmode','on');
      | port_label(ports(4).type,ports(4).port,ports(4).txt,'texmode','on');
      | port_label(ports(5).type,ports(5).port,ports(5).txt,'texmode','on');
      | port_label(ports(6).type,ports(6).port,ports(6).txt,'texmode','on');
      | port_label(ports(7).type,ports(7).port,ports(7).txt,'texmode','on');
  Bus Selector4 : BusSelector  OutputSignals=Qdyn,alpha,beta
  Demux : Demux  Outputs=[3 3]
  Demux1 : Demux  Outputs=[3 3]
  Direction Cosine Matrix Body to Wind : aerolibtransform2/Direction Cosine Matrix Body to Wind
  Ground : Ground
  Ground1 : Ground
  Manual Switch : ManualSwitch
  Mux : Mux  Inputs=2
  Product : Product  RndMeth=Zero
  Product1 : Product  RndMeth=Zero
  Product2 : Product  Multiplication=Matrix(*)  RndMeth=Zero
  Sum : Sum  Inputs=++|  SaturateOnIntegerOverflow=on  InputSameDT=on  OutDataTypeStr=Inherit: Same as first input
  Terminator : Terminator
  Terminator1 : Terminator
  Terminator2 : Terminator
  To Workspace : ToWorkspace  VariableName=qbar  SampleTime=sampleVec  SaveFormat=Structure With Time
  To Workspace1 : ToWorkspace  VariableName=engineForcesBody  SampleTime=sampleVec  SaveFormat=Structure With Time
  To Workspace2 : ToWorkspace  VariableName=aeroForcesBody  SampleTime=-1  SaveFormat=Structure With Time
  To Workspace3 : ToWorkspace  VariableName=aeroForcesWind  SampleTime=-1  SaveFormat=Structure With Time
  neglect center of gravity  and center of pressure effects : Constant  Value=[0 0 0]
  reference area : Gain  Gain=beaver_S  SaturateOnIntegerOverflow=on  OutDataTypeStr=Inherit: Same as input  ParamDataTypeStr=Inherit: Same as input
  reference area1 : Gain  Gain=beaver_S  SaturateOnIntegerOverflow=on  OutDataTypeStr=Inherit: Same as input  ParamDataTypeStr=Inherit: Same as input
  XYZ : Outport
  LMN : Outport  Port=2
  wires:
  Sum/1 -> Aerodynamic Forces and Moments/1(Coefficients)
  Aero Coefficients/1 -> Sum/2, Demux/1
  Aerodynamic Forces and Moments/2(Moments) -> LMN/1
  Fltparams/1 -> Bus Selector4/1
  Aerodynamic Forces and Moments/1(Forces) -> XYZ/1
  neglect center of gravity  and center of pressure effects/1 -> Aerodynamic Forces and Moments/4(CP), Aerodynamic Forces and Moments/3(CG)
  Bus Selector4/1 -> To Workspace/1, Aerodynamic Forces and Moments/2(qbar), Product/2, Product1/1  "<Qdyn>"
  Bus Selector4/2 -> Mux/1  "<alpha>"
  Bus Selector4/3 -> Mux/2  "<beta>"
  reference area/1 -> Product/1
  reference area1/1 -> Product1/2
  Product1/1 -> To Workspace2/1, Product2/2
  Mux/1 -> Direction Cosine Matrix Body to Wind/1
  Direction Cosine Matrix Body to Wind/1 -> Product2/1
  Product2/1 -> To Workspace3/1
  Demux/2 -> Terminator/1
  Demux/1 -> reference area1/1
  Engine Coefficients/1 -> Terminator1/1
  Demux1/1 -> reference area/1
  Demux1/2 -> Terminator2/1
  Manual Switch/1 -> To Workspace1/1
  Product/1 -> Manual Switch/1
  Ground1/1 -> Manual Switch/2
  Ground/1 -> Sum/1, Demux1/1

== system asbdhc2/DeHavilland Beaver Airframe/Aircraft Dynamics/Total Forces  and Moments/Gravity  ==
  g : Inport
  DCM : Inport  Port=2
  Gravity in Earth Axes : Gain  Gain=beaver_mass  SaturateOnIntegerOverflow=on  OutDataTypeStr=Inherit: Same as input  ParamDataTypeStr=Inherit: Same as input
  Inertial to Body : Product  Multiplication=Matrix(*)  SaturateOnIntegerOverflow=on  InputSameDT=on  OutDataTypeStr=Inherit: Same as first input
  Reshape : Reshape  OutputDimensionality=Column vector (2-D)
  Reshape1 : Reshape
  Fgrav : Outport
  wires:
  Inertial to Body/1 -> Reshape1/1
  g/1 -> Gravity in Earth Axes/1
  DCM/1 -> Inertial to Body/1
  Gravity in Earth Axes/1 -> Reshape/1
  Reshape/1 -> Inertial to Body/2
  Reshape1/1 -> Fgrav/1

== system asbdhc2/DeHavilland Beaver Airframe/Aircraft Dynamics/Total Forces  and Moments/Aerodynamics/Actuator Increments ==
  alpha : Inport
  beta : Inport  Port=2
  Actuator Deflections : Inport  Port=3
  Aileron : Subsystem
  Elevator : Subsystem
  Flap : Subsystem
  Rudder : Subsystem
  Sum : Sum  Inputs=++++  SaturateOnIntegerOverflow=on  InputSameDT=on  OutDataTypeStr=Inherit: Same as first input
  Coefficients : Outport
  wires:
  Actuator Deflections/1 -> Flap/2(Actuators), Aileron/2(Actuators), Elevator/1(Actuators), Rudder/2(Actuators)
  alpha/1 -> Flap/1(Alpha), Rudder/1(Alpha), Aileron/1(alpha)
  beta/1 -> Elevator/2(Beta)
  Aileron/1(delCoeff) -> Sum/1
  Elevator/1(delCoeff) -> Sum/2
  Rudder/1(delCoeff) -> Sum/3
  Flap/1(delCoeff) -> Sum/4
  Sum/1 -> Coefficients/1
